simulink model "progStateFeedbackIntegralActObsSim"  (R2018b)
settings: Solver=ode45  StartTime=0.0  StopTime=10.0  MaxStep=0.005  RelTol=1e-3  EnableMultiTasking=on
values from neighbouring files (symbols this model uses):
  A = [0 1 0; 0 -1 1; 0 0 -5]    [main.m]
  B = [0 0 5]'    [main.m]
  C = [1 0 0]    [main.m]
  G = Kobs'    [progStateFeedbackIntegralActObs.m]
  KackerMod = -acker(Amod,Bmod,eig_cl_des)    [progStateFeedbackIntegralAct.m]
  n = size(A,1)    [main.m]
  x0 = [2 1 0]    [main.m]
settings Model: Creator=roberto  LastModifiedBy=roberto
settings DataIOCC: LimitDataPoints=on  SaveFormat=Array
settings OptimizationCC: LifeSpan=inf
settings DebuggingCC: SFUnexpectedBacktrackingDiag=warning  SFNoUnconditionalDefaultTransitionDiag=warning  SFExecutionAtInitializationDiag=none
settings HardwareCC: ProdBitPerPointer=32  ProdBitPerSizeT=32  ProdBitPerPtrDiffT=32  ProdLargestAtomicFloat=None  ProdIntDivRoundTo=Undefined  ProdEndianess=Unspecified  ProdWordSize=32  ProdHWDeviceType=32-bit Generic
settings ModelReferenceCC: PropagateSignalLabelsOutOfModel=off
settings SFSimCC: SimUseLocalCustomCode=off
settings RTWCC: RTWUseLocalCustomCode=off
settings CodeAppCC: StateflowObjectComments=on
settings GRTTargetCC: TargetLangStandard=C89/C90 (ANSI)  GeneratePreprocessorConditionals=Disable all
settings ConfigComp: CovMetricSettings=dw  CovHtmlReporting=on  CovSaveCumulativeToWorkspaceVar=on  CovSaveSingleToWorkspaceVar=on  CovExternalEMLEnable=off

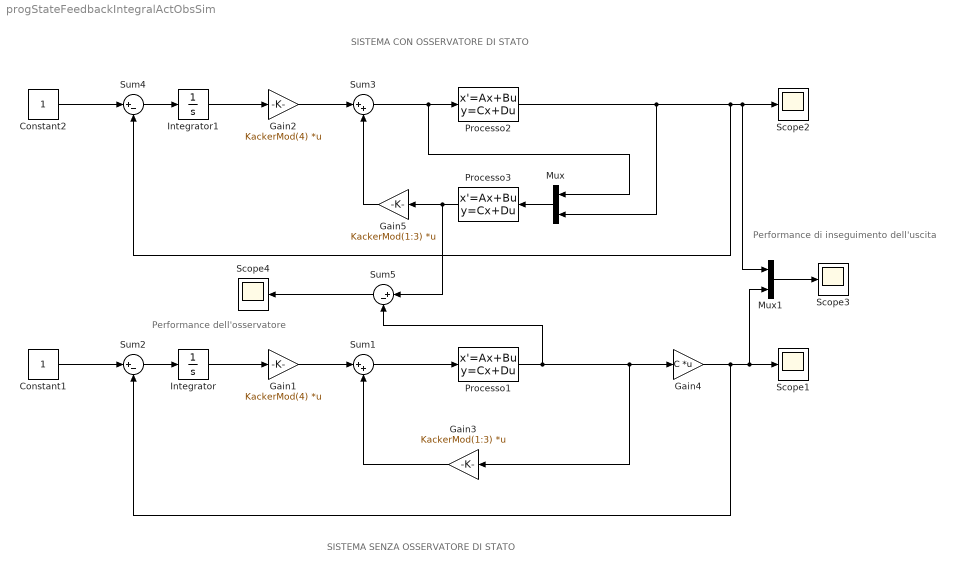
== system progStateFeedbackIntegralActObsSim ==
  note: SISTEMA CON OSSERVATORE DI STATO
  note: SISTEMA SENZA OSSERVATORE DI STATO
  note: Performance di inseguimento dell'uscita
  note: Performance dell'osservatore
  Constant1 : Constant
  Constant2 : Constant
  Gain1 : Gain  Gain=KackerMod(4)  Multiplication=Matrix(K*u)
  Gain2 : Gain  Gain=KackerMod(4)  Multiplication=Matrix(K*u)
  Gain3 : Gain  Gain=KackerMod(1:3)  Multiplication=Matrix(K*u)
  Gain4 : Gain  Gain=C  Multiplication=Matrix(K*u)
  Gain5 : Gain  Gain=KackerMod(1:3)  Multiplication=Matrix(K*u)
  Integrator : Integrator
  Integrator1 : Integrator
  Mux : Mux  Inputs=2
  Mux1 : Mux  Inputs=2
  Processo1 : StateSpace  A=A  B=B  C=eye(n)  D=zeros(n,1)  InitialCondition=x0
  Processo2 : StateSpace  A=A  B=B  C=C  D=0  InitialCondition=x0
  Processo3 : StateSpace  A=A-G*C  B=[B G]  C=eye(3)  D=zeros(3,2)  InitialCondition=x0*0
  Scope{1..4} (4 alike) : Scope
  Sum1 : Sum  Inputs=|++
  Sum2 : Sum  Inputs=|+-
  Sum3 : Sum  Inputs=|++
  Sum4 : Sum  Inputs=|+-
  Sum5 : Sum  Inputs=|+-
  wires:
  Gain4/1 -> Sum2/2, Mux1/2, Scope1/1
  Processo1/1 -> Sum5/2, Gain3/1, Gain4/1
  Gain3/1 -> Sum1/2
  Constant1/1 -> Sum2/1
  Gain1/1 -> Sum1/1
  Sum1/1 -> Processo1/1
  Sum2/1 -> Integrator/1
  Integrator/1 -> Gain1/1
  Processo2/1 -> Mux/2, Sum4/2, Mux1/1, Scope2/1
  Processo3/1 -> Sum5/1, Gain5/1
  Constant2/1 -> Sum4/1
  Sum4/1 -> Integrator1/1
  Integrator1/1 -> Gain2/1
  Gain2/1 -> Sum3/1
  Sum3/1 -> Mux/1, Processo2/1
  Mux/1 -> Processo3/1
  Mux1/1 -> Scope3/1
  Gain5/1 -> Sum3/2
  Sum5/1 -> Scope4/1
